simulink model "VIENA_part4"  (R2024b)
settings: Solver=VariableStepAuto  StartTime=0.0  StopTime=t_max  FixedStep=dt  MaxStep=1e-4  RelTol=1e-4
values from neighbouring files (symbols this model uses):
  A = carParameters.frontalArea    [run.m]
  Cd = carParameters.dragCoefficient    [run.m]
  equivalentMass = ((carParameters.Mass) + (totalInertia/(carParameters.wheelRadius^2)))    [run.m]
  fr = carParameters.wheelFriction    [run.m]
  g = 9.81    [run.m]
  lf = 3.23/2    (= 1.615)    [run.m]
  LM = 1.0122e-3    (= 0.0010122)    [run.m]
  LMatrix = [LS 0 LM 0; 0 LS 0 LM; LM 0 LR 0; 0 LM 0 LR]    [run.m]
  lr = 0.06709e-3    (= 6.709e-05)    [run.m]
  LR = lr + LM    (= 0.00107929)    [run.m]
  m = 700 + str2double(mechInput{1})    [run.m]
  maxID = sqrt(2)*Imb    [run.m]
  maxIQ = sqrt(2*Ib^2 - Imb^2)    [run.m]
  maxTorque = 65    [run.m]
  Pp = 2    [run.m]
  psi0 = atan2((x2-x0),(y2-y0))    [run.m]
  rho = carParameters.airDensity    [run.m]
  RLInv = RMatrix/(LMatrix)    [run.m]
  roadAngle = str2double(mechInput{2})*pi/180    [run.m]
  Rr = 2*5.10e-3    (= 0.0102)    [run.m]
  rw = 0.1651    [run.m]
  Steering = FIAT.SteeringController('method','pure pursuit')    [run.m]
  t_sample = 0.1    [run.m]
  x0 = Map.map_points(1,1)    [run.m]
  y0 = Map.map_points(1,2)    [run.m]
libraries: slpidlib x3, simulink_extras x1, spsEdgeDetectorLib x1, simulink x1
settings Model: Creator=João Fernandes  LastModifiedBy=rafae
settings SolverCC: AlgebraicLoopSolver=TrustRegion
settings DataIOCC: ReturnWorkspaceOutputs=off
settings DebuggingCC: UnconnectedInputMsg=warning  UnconnectedOutputMsg=warning  UnconnectedLineMsg=warning  ArithmeticOperatorsInVariantConditions=warning
settings ModelReferenceCC: EnableRefExpFcnMdlSchedulingChecks=on
settings SFSimCC: SimUseLocalCustomCode=off  CustomCodeUndefinedFunction=UseInterfaceOnly
settings RTWCC: RTWUseLocalCustomCode=off  GPUComputeCapability=3.5

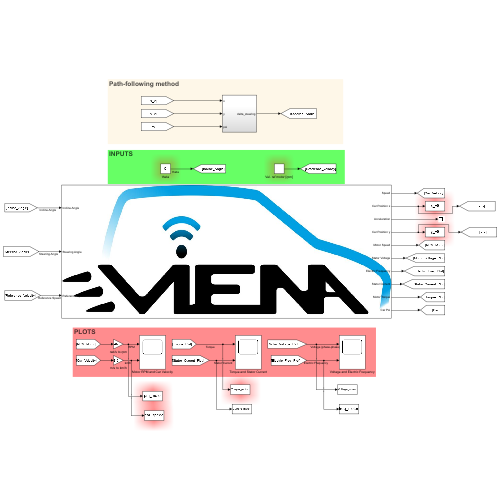
[thumbnail: Simulink's stored preview of the top-level diagram]
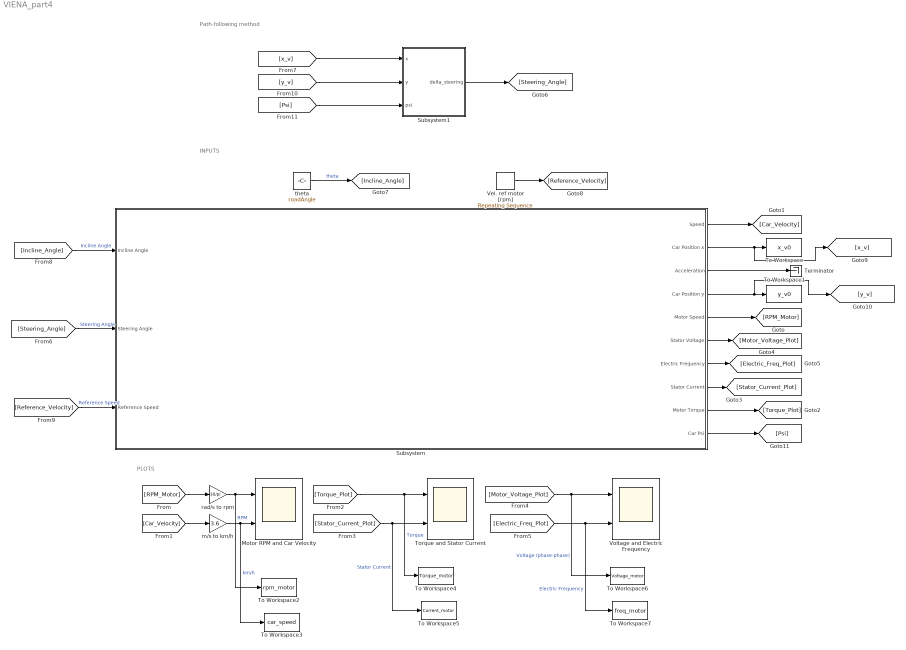
== system VIENA_part4 ==
  note: INPUTS
  note: PLOTS
  note: Path-following method
  Motor RPM and Car Velocity : Scope  NumInputPorts=2
  Subsystem : Subsystem
      mask Display: image('vienalogo.jpg');
  Subsystem1 : Subsystem
  Terminator : Terminator
  To Workspace : ToWorkspace  VariableName=x_v0  SaveFormat=Timeseries  SampleTime=t_sample
  To Workspace1 : ToWorkspace  VariableName=y_v0  SaveFormat=Timeseries  SampleTime=t_sample
  To Workspace2 : ToWorkspace  VariableName=rpm_motor  SaveFormat=Timeseries  SampleTime=t_sample
  To Workspace3 : ToWorkspace  VariableName=car_speed  SaveFormat=Timeseries  SampleTime=t_sample
  To Workspace4 : ToWorkspace  VariableName=Torque_motor  SaveFormat=Timeseries  SampleTime=t_sample
  To Workspace5 : ToWorkspace  VariableName=Current_motor  SaveFormat=Timeseries  SampleTime=-1
  To Workspace6 : ToWorkspace  VariableName=Voltage_motor  SaveFormat=Timeseries  SampleTime=-1
  To Workspace7 : ToWorkspace  VariableName=freq_motor  SaveFormat=Timeseries  SampleTime=-1
  Torque and Stator Current : Scope  NumInputPorts=2
  Vel. ref motor [rpm] : simulink/Sources/Repeating Sequence  rep_seq_t=v_t  rep_seq_y=v_v
  Voltage and Electric Frequency : Scope  NumInputPorts=2
  m/s to km/h : Gain  Gain=3.6
  rad/s to rpm : Gain  Gain=30/pi
  theta : Constant  Value=roadAngle
  wires:
  [RPM_Motor] -> rad/s to rpm/1
  [Car_Velocity] -> m/s to km/h/1
  m/s to km/h/1 -> To Workspace3/1, Motor RPM and Car Velocity/2  "km/h"
  rad/s to rpm/1 -> To Workspace2/1, Motor RPM and Car Velocity/1  "RPM"
  [Torque_Plot] -> To Workspace4/1, Torque and Stator Current/1  "Torque"
  [Stator_Current_Plot] -> To Workspace5/1, Torque and Stator Current/2  "Stator Current"
  [Motor_Voltage_Plot] -> To Workspace6/1, Voltage and Electric Frequency/1  "Voltage (phase-phase)"
  [Electric_Freq_Plot] -> To Workspace7/1, Voltage and Electric Frequency/2  "Electric Frequency"
  theta/1 -> [Incline_Angle]  "theta"
  Vel. ref motor [rpm]/1 -> [Reference_Velocity]
  [Incline_Angle] -> Subsystem/1(Incline Angle)  "Incline Angle"
  [Steering_Angle] -> Subsystem/2(Steering Angle)  "Steering Angle"
  [Reference_Velocity] -> Subsystem/3(Reference Speed)  "Reference Speed"
  Subsystem/1(Speed) -> [Car_Velocity]
  Subsystem/2(Car Position x) -> [x_v], To Workspace/1
  Subsystem/3(Acceleration) -> Terminator/1
  Subsystem/4(Car Position y) -> [y_v], To Workspace1/1
  Subsystem/5(Motor Speed) -> [RPM_Motor]
  Subsystem/6(Stator Voltage) -> [Motor_Voltage_Plot]
  Subsystem/7(Electric Frequency) -> [Electric_Freq_Plot]
  Subsystem/8(Stator Current) -> [Stator_Current_Plot]
  Subsystem/9(Motor Torque) -> [Torque_Plot]
  [x_v] -> Subsystem1/1(x)
  [y_v] -> Subsystem1/2(y)
  Subsystem1/1(delta_steering) -> [Steering_Angle]
  Subsystem/10(Car Psi) -> [Psi]
  [Psi] -> Subsystem1/3(psi)

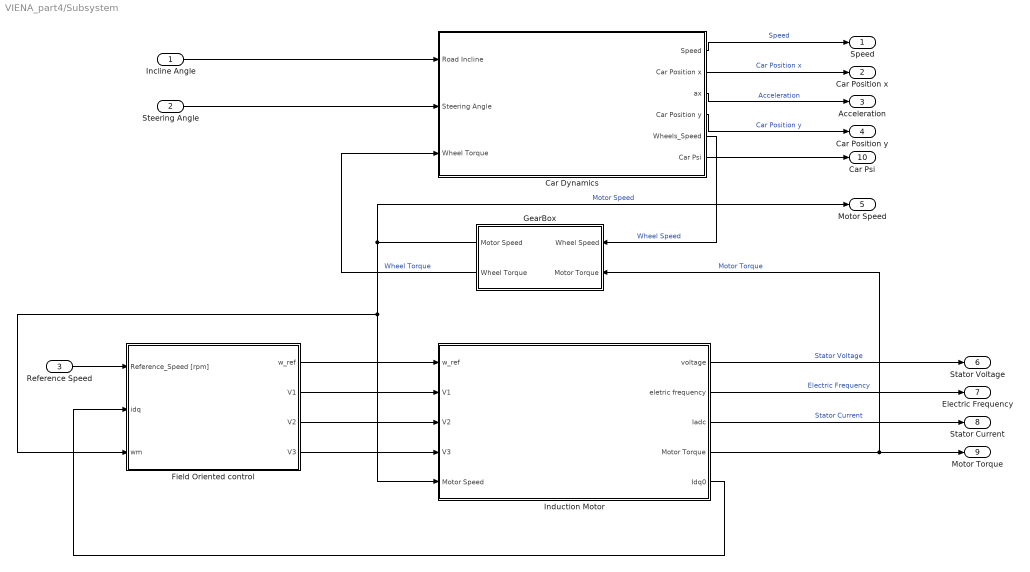
== system VIENA_part4/Subsystem ==
  Incline Angle : Inport
  Steering Angle : Inport  Port=2
  Reference Speed : Inport  Port=3
  Car Dynamics : Subsystem
  "Field Oriented control " : Subsystem
  GearBox : Subsystem
  Induction Motor : Subsystem
  Speed : Outport  VectorParamsAs1DForOutWhenUnconnected=off
  Car Position x : Outport  Port=2  VectorParamsAs1DForOutWhenUnconnected=off
  Acceleration : Outport  Port=3  VectorParamsAs1DForOutWhenUnconnected=off
  Car Position y : Outport  Port=4  VectorParamsAs1DForOutWhenUnconnected=off
  Motor Speed : Outport  Port=5  VectorParamsAs1DForOutWhenUnconnected=off
  Stator Voltage : Outport  Port=6  VectorParamsAs1DForOutWhenUnconnected=off
  Electric Frequency : Outport  Port=7  VectorParamsAs1DForOutWhenUnconnected=off
  Stator Current : Outport  Port=8  VectorParamsAs1DForOutWhenUnconnected=off
  Motor Torque : Outport  Port=9  VectorParamsAs1DForOutWhenUnconnected=off
  Car Psi : Outport  Port=10  VectorParamsAs1DForOutWhenUnconnected=off
  wires:
  GearBox/1("Motor Speed ") -> Induction Motor/5(Motor Speed), "Field Oriented control "/3(wm), Motor Speed/1  "Motor Speed"
  GearBox/2(Wheel Torque) -> Car Dynamics/3(Wheel Torque)  "Wheel Torque"
  Incline Angle/1 -> Car Dynamics/1(Road Incline)
  Induction Motor/1(voltage) -> Stator Voltage/1  "Stator Voltage"
  Car Dynamics/1(Speed) -> Speed/1  "Speed"
  Car Dynamics/5(Wheels_Speed) -> GearBox/1(Wheel Speed)  "Wheel Speed"
  Induction Motor/2(eletric frequency) -> Electric Frequency/1  "Electric Frequency"
  Induction Motor/4(Motor Torque) -> Motor Torque/1, GearBox/2(Motor Torque)  "Motor Torque"
  Car Dynamics/2(Car Position x) -> Car Position x/1  "Car Position x"
  Steering Angle/1 -> Car Dynamics/2(Steering Angle)
  Car Dynamics/4(Car Position y) -> Car Position y/1  "Car Position y"
  Induction Motor/3(Iadc) -> Stator Current/1  "Stator Current"
  Car Dynamics/3(ax) -> Acceleration/1  "Acceleration"
  Car Dynamics/6(Car Psi) -> Car Psi/1
  Reference Speed/1 -> "Field Oriented control "/1(Reference_Speed [rpm])
  "Field Oriented control "/2(V1) -> Induction Motor/2(V1)
  "Field Oriented control "/1(w_ref) -> Induction Motor/1(w_ref)
  "Field Oriented control "/3(V2) -> Induction Motor/3(V2)
  "Field Oriented control "/4(V3) -> Induction Motor/4(V3)
  Induction Motor/5(Idq0) -> "Field Oriented control "/2(idq)

== system VIENA_part4/Subsystem1 ==
  x : Inport
  y : Inport  Port=2
  psi : Inport  Port=3
  Clock : simulink_extras/Flip Flops/Clock  period=dt
  Control steering (with fixed frequency) : Subsystem  TreatAsAtomicUnit=on
  Edge Detector1 : spsEdgeDetectorLib/Edge Detector  model=Rising  ic=0  Ts=0
      settings: LibrarySourceBlock=sps_lib/Control/Edge Detector
  Memory : Memory
  Scope : Scope  NumInputPorts=3
  delta_steering : Outport  VectorParamsAs1DForOutWhenUnconnected=off
  wires:
  Edge Detector1/1 -> Control steering (with fixed frequency)/Enable, Scope/2
  Clock/1 -> Edge Detector1/1
  x/1 -> Control steering (with fixed frequency)/1(x)
  y/1 -> Control steering (with fixed frequency)/2(y)
  psi/1 -> Control steering (with fixed frequency)/3(psi)
  Control steering (with fixed frequency)/1(delta) -> Memory/1, Scope/1
  Memory/1 -> Scope/3, delta_steering/1

== system VIENA_part4/Subsystem/Car Dynamics ==
  Road Incline : Inport
  Steering Angle : Inport  Port=2
  Wheel Torque : Inport  Port=3
  Car Position : Subsystem
  x-simplified model vehicle+wheel : Subsystem
  Speed : Outport  VectorParamsAs1DForOutWhenUnconnected=off
  Car Position x : Outport  Port=2  VectorParamsAs1DForOutWhenUnconnected=off
  ax : Outport  Port=3  VectorParamsAs1DForOutWhenUnconnected=off
  Car Position y : Outport  Port=4  VectorParamsAs1DForOutWhenUnconnected=off
  Wheels_Speed : Outport  Port=5  VectorParamsAs1DForOutWhenUnconnected=off
  Car Psi : Outport  Port=6  VectorParamsAs1DForOutWhenUnconnected=off
  wires:
  Wheel Torque/1 -> x-simplified model vehicle+wheel/1(wheel_Torque)
  x-simplified model vehicle+wheel/1(Speed) -> Speed/1, Car Position/3(Speed)
  x-simplified model vehicle+wheel/2(Acceleration) -> ax/1  "ax"
  Steering Angle/1 -> Car Position/1(Steering Angle)
  Car Position/2(Car Position y) -> Car Position y/1  "Car_Position_y"
  Road Incline/1 -> x-simplified model vehicle+wheel/2(Incline Angle), Car Position/2(Road Incline)
  x-simplified model vehicle+wheel/3(Wheels_Speed) -> Wheels_Speed/1
  Car Position/1(Car Position x) -> Car Position x/1  "Car_Position_x"
  Car Position/3(Car psi) -> Car Psi/1

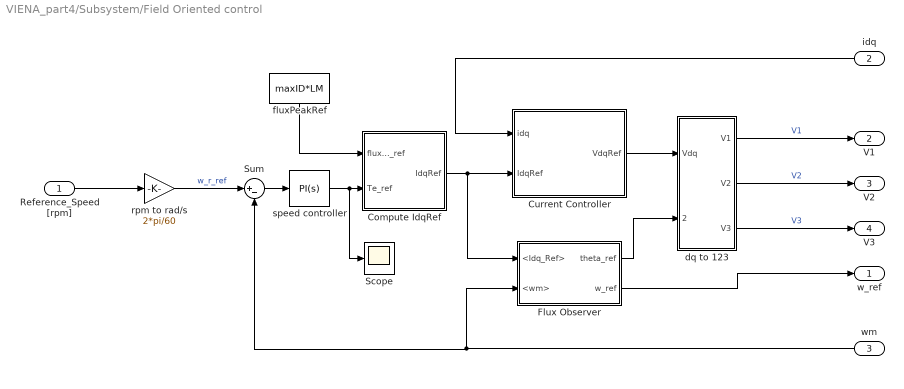
== system VIENA_part4/Subsystem/Field Oriented control  ==
  Reference_Speed [rpm] : Inport
  idq : Inport  Port=2
  wm : Inport  Port=3
  Compute IdqRef : Subsystem
  Current Controller : Subsystem
  Flux Observer : Subsystem
  Scope : Scope
  Sum : Sum  Inputs=|+-
  dq to 123 : Subsystem
  fluxPeakRef : Constant  Value=maxID*LM
  rpm to rad/s : Gain  Gain=2*pi/60
  speed controller : slpidlib/PID Controller  Controller=PI  Form=Parallel  TimeDomain=Continuous-time  UseExternalTs=off  SampleTime=-1  IntegratorMethod=Forward Euler  FilterMethod=Forward Euler  ControllerParametersSource=internal  P=50  I=100  UseKiTs=off  D=0  UseExternalDerivativeSource=off  N=100  UseFilter=on  TunerSelectOption=Transfer Function Based (PID Tuner App)  InitialConditionSource=internal  InitialConditionForIntegrator=0  InitialConditionForFilter=0  DifferentiatorICPrevScaledInput=0  ExternalReset=none  TrackingMode=off  Kt=1  LimitOutput=on  SatLimitsSource=internal  UpperSaturationLimit=maxTorque  LowerSaturationLimit=-maxTorque  LinearizeAsGain=on  AntiWindupMode=back-calculation  Kb=500  LimitIntegrator=off  UpperIntegratorSaturationLimit=inf  LowerIntegratorSaturationLimit=-inf  POutMin=[]  POutMax=[]  IOutMin=[]  IOutMax=[]  DOutMin=[]  DOutMax=[]  NOutMin=[]  NOutMax=[]  SumOutMin=[]  SumOutMax=[]  SaturationOutMin=[]  SaturationOutMax=[]  PParamMin=[]  PParamMax=[]  IParamMin=[]  IParamMax=[]  DParamMin=[]  DParamMax=[]  NParamMin=[]  NParamMax=[]  KbParamMin=[]  KbParamMax=[]  KtParamMin=[]  KtParamMax=[]  KbOutMin=[]  KbOutMax=[]  KtOutMin=[]  KtOutMax=[]  IntegratorOutMin=[]  IntegratorOutMax=[]  FilterOutMin=[]  FilterOutMax=[]  SumI1OutMin=[]  SumI1OutMax=[]  SumI2OutMin=[]  SumI2OutMax=[]  SumI3OutMin=[]  SumI3OutMax=[]  SumI4OutMin=[]  SumI4OutMax=[]  SumDOutMin=[]  SumDOutMax=[]  DifferentiatorOutMin=[]  DifferentiatorOutMax=[]  FilterDiffOutCoefMin=[]  FilterDiffOutCoefMax=[]  ReciprocalOutMin=[]  ReciprocalOutMax=[]  SumDenOutMin=[]  SumDenOutMax=[]  SumNumOutMin=[]  SumNumOutMax=[]  DivideOutMin=[]  DivideOutMax=[]  UdiffTsProdOutMin=[]  UdiffTsProdOutMax=[]  NTsProdOutMin=[]  NTsProdOutMax=[]  UintegralTsProdOutMin=[]  UintegralTsProdOutMax=[]  UngainTsProdOutMin=[]  UngainTsProdOutMax=[]  ClampingZeroOutDataTypeStr=Inherit: Inherit via back propagation  ClampingZeroOutMin=[]  ClampingZeroOutMax=[]  FilterDenConstantOutDataTypeStr=Inherit: Inherit via back propagation  FilterDenConstantOutMin=[]  FilterDenConstantOutMax=[]  PCopyOutDataTypeStr=Inherit: Inherit via back propagation  PCopyOutMin=[]  PCopyOutMax=[]  NCopyOutDataTypeStr=Inherit: Inherit via back propagation  NCopyOutMin=[]  NCopyOutMax=[]  IntegratorContinuousStateAttributes=''  IntegratorStateMustResolveToSignalObject=off  IntegratorRTWStateStorageClass=Auto  FilterContinuousStateAttributes=''  FilterStateMustResolveToSignalObject=off  FilterRTWStateStorageClass=Auto  ParallelPVariant=InternalParameters  IdealPVariant=Disabled  IVariant=InternalParameters  DVariant=Disabled  IntegratorVariant=Continuous  SatVariant=Enabled  AWVariant=BackCalculation  PCopyVariant=Disabled  TRVariant=Disabled  FdbkBlocksVariant=Forward  IdealPFdbkVariant=Disabled  SatFdbkVariant=Disabled  DerivativeFilterVariant=Disabled  NVariant=Disabled  NCopyVariant=Disabled_SignalSpec  FilterICVariant=Disabled  IntegratorICVariant=InternalICs  ExternalResetVariant=Disabled  TRSumVariant=Passthrough  SumFdbkVariant=Disabled  SumVariant=Sum_PI  TsampFilterVariant=InternalTs  TsampNgainVariant=Passthrough  TsampIntegralVariant=Disabled_SignalSpec  ExternalSaturationOutDataTypeStr=Inherit: Same as second input  DerivativeSourceVariant=Disabled  PreIntVariant=InternalPreInt
  w_ref : Outport  VectorParamsAs1DForOutWhenUnconnected=off
  V1 : Outport  Port=2  VectorParamsAs1DForOutWhenUnconnected=off
  V2 : Outport  Port=3  VectorParamsAs1DForOutWhenUnconnected=off
  V3 : Outport  Port=4  VectorParamsAs1DForOutWhenUnconnected=off
  wires:
  wm/1 -> Sum/2, Flux Observer/2(<wm>)
  Current Controller/1(VdqRef) -> dq to 123/1(Vdq)
  idq/1 -> Current Controller/1(idq)
  Flux Observer/2(w_ref) -> w_ref/1
  Compute IdqRef/1(IdqRef) -> Flux Observer/1(<Idq_Ref>), Current Controller/2(IdqRef)
  Sum/1 -> speed controller/1
  fluxPeakRef/1 -> Compute IdqRef/1(fluxdR_ref)
  Flux Observer/1(theta_ref) -> dq to 123/2(theta_ref)
  dq to 123/3(V3) -> V3/1  "V3"
  dq to 123/1(V1) -> V1/1  "V1"
  speed controller/1 -> Scope/1, Compute IdqRef/2(Te_ref)
  dq to 123/2(V2) -> V2/1  "V2"
  Reference_Speed [rpm]/1 -> rpm to rad/s/1
  rpm to rad/s/1 -> Sum/1  "w_r_ref"

== system VIENA_part4/Subsystem/GearBox ==
  Wheel Speed : Inport
  Motor Torque : Inport  Port=2
  Gain : Gain  Gain=8
  Gain1 : Gain  Gain=8
  "Motor Speed " : Outport  VectorParamsAs1DForOutWhenUnconnected=off
  Wheel Torque : Outport  Port=2  VectorParamsAs1DForOutWhenUnconnected=off
  wires:
  Wheel Speed/1 -> Gain/1
  Gain/1 -> "Motor Speed "/1
  Motor Torque/1 -> Gain1/1
  Gain1/1 -> Wheel Torque/1

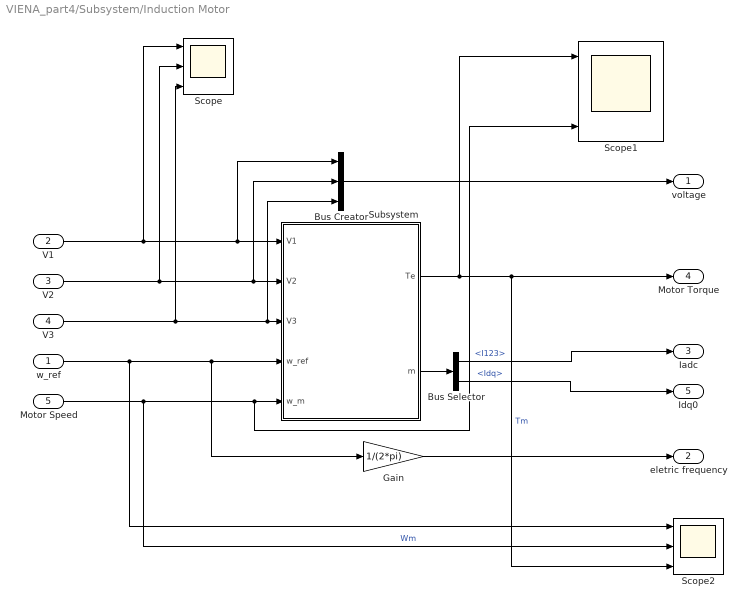
== system VIENA_part4/Subsystem/Induction Motor ==
  w_ref : Inport
  V1 : Inport  Port=2
  V2 : Inport  Port=3
  V3 : Inport  Port=4
  Motor Speed : Inport  Port=5
  Bus Creator : BusCreator  Inputs=3
  Bus Selector : BusSelector  OutputSignals=I123,Idq
  Gain : Gain  Gain=1/(2*pi)
  Scope : Scope  NumInputPorts=3
  Scope1 : Scope  NumInputPorts=3
  Scope2 : Scope  NumInputPorts=3
  Subsystem : Subsystem
  voltage : Outport  VectorParamsAs1DForOutWhenUnconnected=off
  eletric frequency : Outport  Port=2  VectorParamsAs1DForOutWhenUnconnected=off
  Iadc : Outport  Port=3  VectorParamsAs1DForOutWhenUnconnected=off
  Motor Torque : Outport  Port=4  VectorParamsAs1DForOutWhenUnconnected=off
  Idq0 : Outport  Port=5  VectorParamsAs1DForOutWhenUnconnected=off
  wires:
  Subsystem/1(Te) -> Scope1/1, Scope2/3, Motor Torque/1  "Tm"
  Motor Speed/1 -> Scope2/2, Scope1/3, Subsystem/5(w_m)  "Wm"
  Subsystem/2(m) -> Bus Selector/1
  Bus Selector/1 -> Iadc/1  "<I123>"
  V3/1 -> Scope/3, Bus Creator/3, Subsystem/3(V3)
  V2/1 -> Bus Creator/2, Subsystem/2(V2), Scope/2
  V1/1 -> Bus Creator/1, Subsystem/1(V1), Scope/1
  w_ref/1 -> Scope2/1, Gain/1, Subsystem/4(w_ref)
  Gain/1 -> eletric frequency/1
  Bus Creator/1 -> voltage/1
  Bus Selector/2 -> Idq0/1  "<Idq>"

== system VIENA_part4/Subsystem1/Control steering (with fixed frequency) ==
  x : Inport
  y : Inport  Port=2
  psi : Inport  Port=3
  Enable : EnablePort
  Constant1 : Constant  Value=Steering.map_points  VectorParams1D=off
  Saturation : Saturate  UpperLimit=28*pi/180  LowerLimit=-28*pi/180
  Stop Simulation : Stop
  compute diff angle : MATLAB Function  TreatAsAtomicUnit=on
  cria look_ahead : MATLAB Function  TreatAsAtomicUnit=on
  find index : MATLAB Function  TreatAsAtomicUnit=on
  delta : Outport  VectorParamsAs1DForOutWhenUnconnected=off
  wires:
  x/1 -> compute diff angle/2(x), find index/2(x)
  y/1 -> compute diff angle/3("y "), find index/3("y ")
  Constant1/1 -> cria look_ahead/1(map), find index/1(u)
  find index/1(y) -> cria look_ahead/2(path_index)
  cria look_ahead/2(y2) -> Stop Simulation/1
  compute diff angle/1(y) -> Saturation/1
  cria look_ahead/1(y1) -> compute diff angle/1(zone)
  psi/1 -> compute diff angle/4(psi)
  Saturation/1 -> delta/1

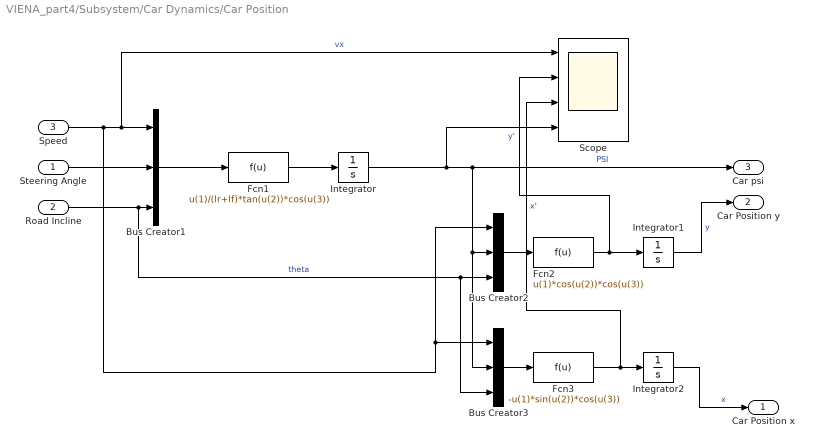
== system VIENA_part4/Subsystem/Car Dynamics/Car Position ==
  Steering Angle : Inport
  Road Incline : Inport  Port=2
  Speed : Inport  Port=3
  Bus Creator1 : BusCreator  Inputs=3
  Bus Creator2 : BusCreator  Inputs=3
  Bus Creator3 : BusCreator  Inputs=3
  Fcn1 : Fcn  Expr=u(1)/(lr+lf)*tan(u(2))*cos(u(3))
  Fcn2 : Fcn  Expr=u(1)*cos(u(2))*cos(u(3))
  Fcn3 : Fcn  Expr=-u(1)*sin(u(2))*cos(u(3))
  Integrator : Integrator  InitialCondition=psi0
  Integrator1 : Integrator  InitialCondition=y0
  Integrator2 : Integrator  InitialCondition=x0
  Scope : Scope  NumInputPorts=4
  Car Position x : Outport  VectorParamsAs1DForOutWhenUnconnected=off
  Car Position y : Outport  Port=2  VectorParamsAs1DForOutWhenUnconnected=off
  Car psi : Outport  Port=3  VectorParamsAs1DForOutWhenUnconnected=off
  wires:
  Integrator1/1 -> Car Position y/1  "y"
  Integrator2/1 -> Car Position x/1  "x"
  Road Incline/1 -> Bus Creator3/3, Bus Creator2/3, Bus Creator1/3  "theta"
  Bus Creator1/1 -> Fcn1/1
  Fcn1/1 -> Integrator/1
  Bus Creator2/1 -> Fcn2/1
  Speed/1 -> Bus Creator2/1, Bus Creator3/1, Scope/1, Bus Creator1/1  "vx"
  Fcn2/1 -> Scope/2, Integrator1/1  "y'"
  Fcn3/1 -> Scope/3, Integrator2/1  "x'"
  Integrator/1 -> Car psi/1, Bus Creator3/2, Bus Creator2/2, Scope/4  "PSI"
  Bus Creator3/1 -> Fcn3/1
  Steering Angle/1 -> Bus Creator1/2

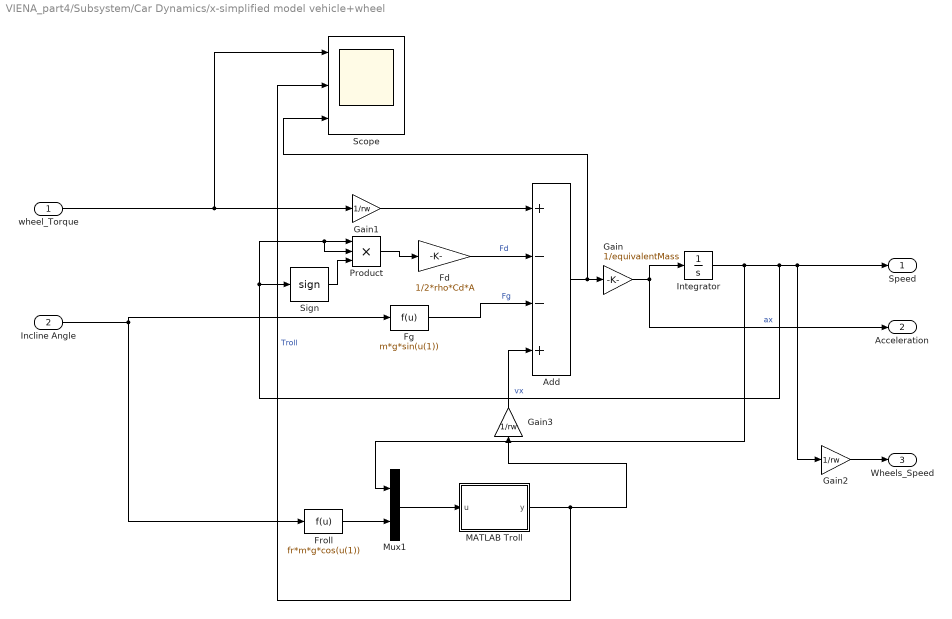
== system VIENA_part4/Subsystem/Car Dynamics/x-simplified model vehicle+wheel ==
  wheel_Torque : Inport
  Incline Angle : Inport  Port=2
  Add : Sum  Inputs=+--+
  Fd : Gain  Gain=1/2*rho*Cd*A
  Fg : Fcn  Expr=m*g*sin(u(1))
  Froll : Fcn  Expr=fr*m*g*cos(u(1))
  Gain : Gain  Gain=1/equivalentMass
  Gain1 : Gain  Gain=1/rw
  Gain2 : Gain  Gain=1/rw
  Gain3 : Gain  Gain=1/rw
  Integrator : Integrator
  MATLAB Troll : MATLAB Function  TreatAsAtomicUnit=on
  Mux1 : Mux  Inputs=2
  Product : Product  Inputs=3
  Scope : Scope  NumInputPorts=3
  Sign : Signum
  Speed : Outport  VectorParamsAs1DForOutWhenUnconnected=off
  Acceleration : Outport  Port=2  VectorParamsAs1DForOutWhenUnconnected=off
  Wheels_Speed : Outport  Port=3  VectorParamsAs1DForOutWhenUnconnected=off
  wires:
  Product/1 -> Fd/1
  Incline Angle/1 -> Froll/1, Fg/1
  Fg/1 -> Add/3  "Fg"
  Add/1 -> Scope/3, Gain/1
  Gain/1 -> Integrator/1, Acceleration/1  "ax"
  Fd/1 -> Add/2  "Fd"
  Integrator/1 -> Mux1/1, Gain2/1, Speed/1, Sign/1, Product/2, Product/1  "vx"
  Sign/1 -> Product/3
  Gain1/1 -> Add/1
  Gain2/1 -> Wheels_Speed/1
  wheel_Torque/1 -> Scope/1, Gain1/1
  Froll/1 -> Mux1/2
  Mux1/1 -> MATLAB Troll/1(u)
  MATLAB Troll/1(y) -> Scope/2, Gain3/1  "Troll"
  Gain3/1 -> Add/4

== system VIENA_part4/Subsystem/Field Oriented control /Compute IdqRef ==
  fluxdR_ref : Inport
  Te_ref : Inport  Port=2
  Fcn : Fcn  Expr=u(2)/(3/2*Pp*(LM/LR)*u(1))
  Gain : Gain  Gain=1/LM
  Mux : Mux  Inputs=2
  Mux1 : Mux  Inputs=2
  Saturation : Saturate  UpperLimit=maxID  LowerLimit=-maxID
  Saturation1 : Saturate  UpperLimit=maxIQ  LowerLimit=-maxIQ
  IdqRef : Outport  VectorParamsAs1DForOutWhenUnconnected=off
  wires:
  fluxdR_ref/1 -> Mux/1, Gain/1
  Mux/1 -> Fcn/1
  Fcn/1 -> Saturation1/1
  Gain/1 -> Saturation/1
  Mux1/1 -> IdqRef/1
  Te_ref/1 -> Mux/2
  Saturation/1 -> Mux1/1  "id"
  Saturation1/1 -> Mux1/2  "iq"

== system VIENA_part4/Subsystem/Field Oriented control /Current Controller ==
  idq : Inport
  IdqRef : Inport  Port=2
  Demux : Demux  Outputs=2
  Mux : Mux  Inputs=2
  PID Controller : slpidlib/PID Controller  Controller=PI  Form=Parallel  TimeDomain=Continuous-time  UseExternalTs=off  SampleTime=-1  IntegratorMethod=Forward Euler  FilterMethod=Forward Euler  ControllerParametersSource=internal  P=5  I=100  UseKiTs=off  D=0  UseExternalDerivativeSource=off  N=100  UseFilter=on  TunerSelectOption=Transfer Function Based (PID Tuner App)  InitialConditionSource=internal  InitialConditionForIntegrator=0  InitialConditionForFilter=0  DifferentiatorICPrevScaledInput=0  ExternalReset=none  TrackingMode=off  Kt=1  LimitOutput=on  SatLimitsSource=internal  UpperSaturationLimit=600  LowerSaturationLimit=-600  LinearizeAsGain=on  AntiWindupMode=back-calculation  Kb=1  LimitIntegrator=off  UpperIntegratorSaturationLimit=inf  LowerIntegratorSaturationLimit=-inf  POutMin=[]  POutMax=[]  IOutMin=[]  IOutMax=[]  DOutMin=[]  DOutMax=[]  NOutMin=[]  NOutMax=[]  SumOutMin=[]  SumOutMax=[]  SaturationOutMin=[]  SaturationOutMax=[]  PParamMin=[]  PParamMax=[]  IParamMin=[]  IParamMax=[]  DParamMin=[]  DParamMax=[]  NParamMin=[]  NParamMax=[]  KbParamMin=[]  KbParamMax=[]  KtParamMin=[]  KtParamMax=[]  KbOutMin=[]  KbOutMax=[]  KtOutMin=[]  KtOutMax=[]  IntegratorOutMin=[]  IntegratorOutMax=[]  FilterOutMin=[]  FilterOutMax=[]  SumI1OutMin=[]  SumI1OutMax=[]  SumI2OutMin=[]  SumI2OutMax=[]  SumI3OutMin=[]  SumI3OutMax=[]  SumI4OutMin=[]  SumI4OutMax=[]  SumDOutMin=[]  SumDOutMax=[]  DifferentiatorOutMin=[]  DifferentiatorOutMax=[]  FilterDiffOutCoefMin=[]  FilterDiffOutCoefMax=[]  ReciprocalOutMin=[]  ReciprocalOutMax=[]  SumDenOutMin=[]  SumDenOutMax=[]  SumNumOutMin=[]  SumNumOutMax=[]  DivideOutMin=[]  DivideOutMax=[]  UdiffTsProdOutMin=[]  UdiffTsProdOutMax=[]  NTsProdOutMin=[]  NTsProdOutMax=[]  UintegralTsProdOutMin=[]  UintegralTsProdOutMax=[]  UngainTsProdOutMin=[]  UngainTsProdOutMax=[]  ClampingZeroOutDataTypeStr=Inherit: Inherit via back propagation  ClampingZeroOutMin=[]  ClampingZeroOutMax=[]  FilterDenConstantOutDataTypeStr=Inherit: Inherit via back propagation  FilterDenConstantOutMin=[]  FilterDenConstantOutMax=[]  PCopyOutDataTypeStr=Inherit: Inherit via back propagation  PCopyOutMin=[]  PCopyOutMax=[]  NCopyOutDataTypeStr=Inherit: Inherit via back propagation  NCopyOutMin=[]  NCopyOutMax=[]  IntegratorContinuousStateAttributes=''  IntegratorStateMustResolveToSignalObject=off  IntegratorRTWStateStorageClass=Auto  FilterContinuousStateAttributes=''  FilterStateMustResolveToSignalObject=off  FilterRTWStateStorageClass=Auto  ParallelPVariant=InternalParameters  IdealPVariant=Disabled  IVariant=InternalParameters  DVariant=Disabled  IntegratorVariant=Continuous  SatVariant=Enabled  AWVariant=BackCalculation  PCopyVariant=Disabled  TRVariant=Disabled  FdbkBlocksVariant=Forward  IdealPFdbkVariant=Disabled  SatFdbkVariant=Disabled  DerivativeFilterVariant=Disabled  NVariant=Disabled  NCopyVariant=Disabled_SignalSpec  FilterICVariant=Disabled  IntegratorICVariant=InternalICs  ExternalResetVariant=Disabled  TRSumVariant=Passthrough  SumFdbkVariant=Disabled  SumVariant=Sum_PI  TsampFilterVariant=InternalTs  TsampNgainVariant=Passthrough  TsampIntegralVariant=Disabled_SignalSpec  ExternalSaturationOutDataTypeStr=Inherit: Same as second input  DerivativeSourceVariant=Disabled  PreIntVariant=InternalPreInt
  PID Controller1 : slpidlib/PID Controller  Controller=PI  Form=Parallel  TimeDomain=Continuous-time  UseExternalTs=off  SampleTime=-1  IntegratorMethod=Forward Euler  FilterMethod=Forward Euler  ControllerParametersSource=internal  P=5  I=100  UseKiTs=off  D=0  UseExternalDerivativeSource=off  N=100  UseFilter=on  TunerSelectOption=Transfer Function Based (PID Tuner App)  InitialConditionSource=internal  InitialConditionForIntegrator=0  InitialConditionForFilter=0  DifferentiatorICPrevScaledInput=0  ExternalReset=none  TrackingMode=off  Kt=1  LimitOutput=on  SatLimitsSource=internal  UpperSaturationLimit=600  LowerSaturationLimit=-600  LinearizeAsGain=on  AntiWindupMode=back-calculation  Kb=1  LimitIntegrator=off  UpperIntegratorSaturationLimit=inf  LowerIntegratorSaturationLimit=-inf  POutMin=[]  POutMax=[]  IOutMin=[]  IOutMax=[]  DOutMin=[]  DOutMax=[]  NOutMin=[]  NOutMax=[]  SumOutMin=[]  SumOutMax=[]  SaturationOutMin=[]  SaturationOutMax=[]  PParamMin=[]  PParamMax=[]  IParamMin=[]  IParamMax=[]  DParamMin=[]  DParamMax=[]  NParamMin=[]  NParamMax=[]  KbParamMin=[]  KbParamMax=[]  KtParamMin=[]  KtParamMax=[]  KbOutMin=[]  KbOutMax=[]  KtOutMin=[]  KtOutMax=[]  IntegratorOutMin=[]  IntegratorOutMax=[]  FilterOutMin=[]  FilterOutMax=[]  SumI1OutMin=[]  SumI1OutMax=[]  SumI2OutMin=[]  SumI2OutMax=[]  SumI3OutMin=[]  SumI3OutMax=[]  SumI4OutMin=[]  SumI4OutMax=[]  SumDOutMin=[]  SumDOutMax=[]  DifferentiatorOutMin=[]  DifferentiatorOutMax=[]  FilterDiffOutCoefMin=[]  FilterDiffOutCoefMax=[]  ReciprocalOutMin=[]  ReciprocalOutMax=[]  SumDenOutMin=[]  SumDenOutMax=[]  SumNumOutMin=[]  SumNumOutMax=[]  DivideOutMin=[]  DivideOutMax=[]  UdiffTsProdOutMin=[]  UdiffTsProdOutMax=[]  NTsProdOutMin=[]  NTsProdOutMax=[]  UintegralTsProdOutMin=[]  UintegralTsProdOutMax=[]  UngainTsProdOutMin=[]  UngainTsProdOutMax=[]  ClampingZeroOutDataTypeStr=Inherit: Inherit via back propagation  ClampingZeroOutMin=[]  ClampingZeroOutMax=[]  FilterDenConstantOutDataTypeStr=Inherit: Inherit via back propagation  FilterDenConstantOutMin=[]  FilterDenConstantOutMax=[]  PCopyOutDataTypeStr=Inherit: Inherit via back propagation  PCopyOutMin=[]  PCopyOutMax=[]  NCopyOutDataTypeStr=Inherit: Inherit via back propagation  NCopyOutMin=[]  NCopyOutMax=[]  IntegratorContinuousStateAttributes=''  IntegratorStateMustResolveToSignalObject=off  IntegratorRTWStateStorageClass=Auto  FilterContinuousStateAttributes=''  FilterStateMustResolveToSignalObject=off  FilterRTWStateStorageClass=Auto  ParallelPVariant=InternalParameters  IdealPVariant=Disabled  IVariant=InternalParameters  DVariant=Disabled  IntegratorVariant=Continuous  SatVariant=Enabled  AWVariant=BackCalculation  PCopyVariant=Disabled  TRVariant=Disabled  FdbkBlocksVariant=Forward  IdealPFdbkVariant=Disabled  SatFdbkVariant=Disabled  DerivativeFilterVariant=Disabled  NVariant=Disabled  NCopyVariant=Disabled_SignalSpec  FilterICVariant=Disabled  IntegratorICVariant=InternalICs  ExternalResetVariant=Disabled  TRSumVariant=Passthrough  SumFdbkVariant=Disabled  SumVariant=Sum_PI  TsampFilterVariant=InternalTs  TsampNgainVariant=Passthrough  TsampIntegralVariant=Disabled_SignalSpec  ExternalSaturationOutDataTypeStr=Inherit: Same as second input  DerivativeSourceVariant=Disabled  PreIntVariant=InternalPreInt
  Scope2 : Scope  NumInputPorts=2
  Sum1 : Sum  Inputs=+-
  VdqRef : Outport  VectorParamsAs1DForOutWhenUnconnected=off
  wires:
  IdqRef/1 -> Scope2/1, Sum1/1
  idq/1 -> Sum1/2
  PID Controller/1 -> Mux/1  "PI"
  Sum1/1 -> Scope2/2, Demux/1  "error"
  Demux/1 -> PID Controller/1
  Demux/2 -> PID Controller1/1
  PID Controller1/1 -> Mux/2
  Mux/1 -> VdqRef/1

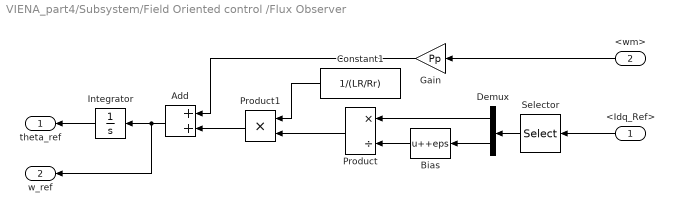
== system VIENA_part4/Subsystem/Field Oriented control /Flux Observer ==
  <Idq_Ref> : Inport
  <wm> : Inport  Port=2
  Add : Sum  Inputs=2
  Bias : Bias  Bias=+eps  SaturateOnIntegerOverflow=off
  Constant1 : Constant  Value=1/(LR/Rr)
  Demux : Demux  Outputs=2
  Gain : Gain  Gain=Pp
  Integrator : Integrator
  Product : Product  Inputs=*/
  Product1 : Product
  Selector : Selector  InputPortWidth=2  IndexOptions=Index vector (dialog)  Indices=[2 1]  OutputSizes=1
  theta_ref : Outport  VectorParamsAs1DForOutWhenUnconnected=off
  w_ref : Outport  Port=2  VectorParamsAs1DForOutWhenUnconnected=off
  wires:
  Demux/1 -> Product/1
  <wm>/1 -> Gain/1
  Constant1/1 -> Product1/1
  Selector/1 -> Demux/1
  Product1/1 -> Add/2
  Product/1 -> Product1/2
  <Idq_Ref>/1 -> Selector/1
  Add/1 -> w_ref/1, Integrator/1
  Bias/1 -> Product/2
  Demux/2 -> Bias/1
  Integrator/1 -> theta_ref/1
  Gain/1 -> Add/1

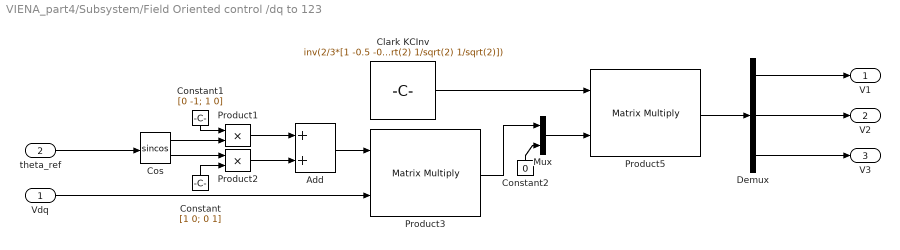
== system VIENA_part4/Subsystem/Field Oriented control /dq to 123 ==
  Vdq : Inport
  theta_ref : Inport  Port=2
  Add : Sum
  Clark KCInv : Constant  Value=inv(2/3*[1 -0.5 -0.5; 0 sqrt(3)/2 -sqrt(3)/2; 1/sqrt(2) 1/sqrt(2) 1/sqrt(2)])
  Constant : Constant  Value=[1 0; 0 1]
  Constant1 : Constant  Value=[0 -1; 1 0]
  Constant2 : Constant  Value=0
  Cos : Trigonometry  Operator=sincos
  Demux : Demux  Outputs=3
  Mux : Mux  Inputs=2
  Product1 : Product
  Product2 : Product
  Product3 : Product  Multiplication=Matrix(*)
  Product5 : Product  Multiplication=Matrix(*)
  V1 : Outport  VectorParamsAs1DForOutWhenUnconnected=off
  V2 : Outport  Port=2  VectorParamsAs1DForOutWhenUnconnected=off
  V3 : Outport  Port=3  VectorParamsAs1DForOutWhenUnconnected=off
  wires:
  Cos/1 -> Product1/2
  Constant1/1 -> Product1/1
  Product2/1 -> Add/2
  Cos/2 -> Product2/1
  Product1/1 -> Add/1
  Constant/1 -> Product2/2
  Add/1 -> Product3/1
  Product3/1 -> Mux/1
  Clark KCInv/1 -> Product5/1
  Mux/1 -> Product5/2
  Constant2/1 -> Mux/2
  Vdq/1 -> Product3/2
  Demux/1 -> V1/1
  Demux/2 -> V2/1
  Demux/3 -> V3/1
  Product5/1 -> Demux/1
  theta_ref/1 -> Cos/1

== system VIENA_part4/Subsystem/Induction Motor/Subsystem ==
  note: V1 - phase-to-neutral voltage of phase 1 [V]
      | V2 - phase-to-neutral voltage of phase 2 [V]
      | V3 - phase-to-neutral voltage of phase 3 [V]
      | w_ref - reference of dq transformation (synchornous electric speed in this case = 2*pi*f) [rad/s]
      | w_m - motor angular speed [rad/s]
  V1 : Inport
  V2 : Inport  Port=2
  V3 : Inport  Port=3
  w_ref : Inport  Port=4
  w_m : Inport  Port=5
  Induction Machine Model : Subsystem
  Te : Outport  VectorParamsAs1DForOutWhenUnconnected=off
  m : Outport  Port=2  VectorParamsAs1DForOutWhenUnconnected=off
  wires:
  Induction Machine Model/1(m) -> m/1
  w_ref/1 -> Induction Machine Model/5(w_ref)
  V1/1 -> Induction Machine Model/2(V1)
  Induction Machine Model/2(Te) -> Te/1
  V2/1 -> Induction Machine Model/3(V2)
  V3/1 -> Induction Machine Model/4(V3)
  w_m/1 -> Induction Machine Model/1(wm)

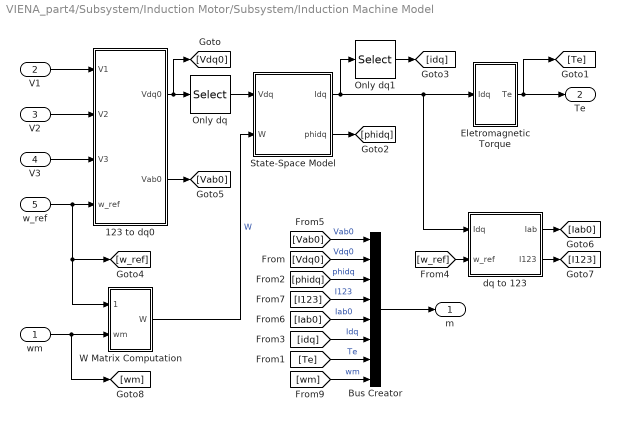
== system VIENA_part4/Subsystem/Induction Motor/Subsystem/Induction Machine Model ==
  wm : Inport
  V1 : Inport  Port=2
  V2 : Inport  Port=3
  V3 : Inport  Port=4
  w_ref : Inport  Port=5
  123 to dq0 : Subsystem
  Bus Creator : BusCreator  Inputs=8
  Eletromagnetic Torque : Subsystem
  Only dq : Selector  InputPortWidth=3  IndexOptions=Index vector (dialog)  Indices=[1 2]  OutputSizes=1
  Only dq1 : Selector  InputPortWidth=4  IndexOptions=Index vector (dialog)  Indices=[1 2]  OutputSizes=1
  State-Space Model : Subsystem
  W Matrix Computation : Subsystem
  dq to 123 : Subsystem
  m : Outport  VectorParamsAs1DForOutWhenUnconnected=off
  Te : Outport  Port=2  VectorParamsAs1DForOutWhenUnconnected=off
  wires:
  123 to dq0/1(Vdq0) -> Only dq/1, [Vdq0]
  V3/1 -> 123 to dq0/3(V3)
  V2/1 -> 123 to dq0/2(V2)
  wm/1 -> [wm], W Matrix Computation/2(wm)
  123 to dq0/2(Vab0) -> [Vab0]
  W Matrix Computation/1(W) -> State-Space Model/2(W)  "W"
  Only dq/1 -> State-Space Model/1(Vdq)
  Eletromagnetic Torque/1(Te) -> Te/1, [Te]
  V1/1 -> 123 to dq0/1(V1)
  State-Space Model/1(Idq) -> dq to 123/1(Idq), Eletromagnetic Torque/1(Idq), Only dq1/1
  [w_ref] -> dq to 123/2(w_ref)
  State-Space Model/2(phidq) -> [phidq]
  dq to 123/1(Iab) -> [Iab0]
  dq to 123/2(I123) -> [I123]
  [Vab0] -> Bus Creator/1  "Vab0"
  [Vdq0] -> Bus Creator/2  "Vdq0"
  [phidq] -> Bus Creator/3  "phidq"
  [I123] -> Bus Creator/4  "I123"
  [Iab0] -> Bus Creator/5  "Iab0"
  [idq] -> Bus Creator/6  "Idq"
  [Te] -> Bus Creator/7  "Te"
  Bus Creator/1 -> m/1
  Only dq1/1 -> [idq]
  w_ref/1 -> 123 to dq0/4(w_ref), W Matrix Computation/1(w_ref), [w_ref]
  [wm] -> Bus Creator/8  "wm"

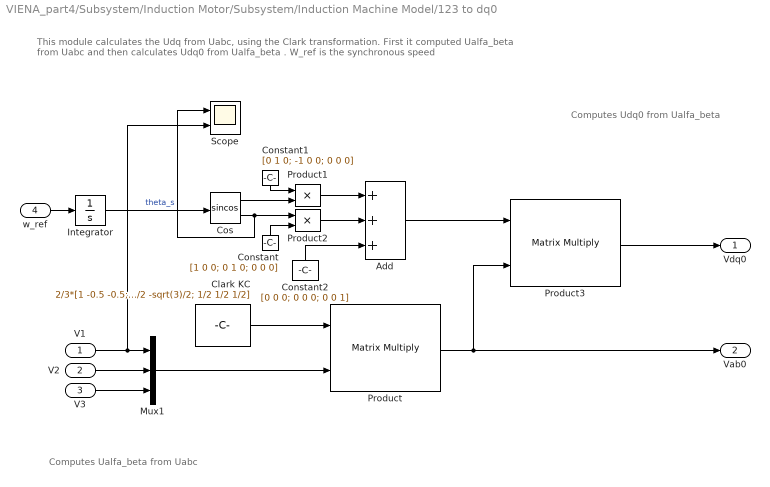
== system VIENA_part4/Subsystem/Induction Motor/Subsystem/Induction Machine Model/123 to dq0 ==
  note: Computes Ualfa_beta from Uabc
  note: This module calculates the Udq from Uabc, using the Clark transformation.
      | First it computed Ualfa_beta from Uabc and then calculates Udq0 from Ualfa_beta .
      | W_ref is the synchronous speed
  note: Computes Udq0 from Ualfa_beta
  V1 : Inport
  V2 : Inport  Port=2
  V3 : Inport  Port=3
  w_ref : Inport  Port=4
  Add : Sum  Inputs=+++
  Clark KC : Constant  Value=2/3*[1 -0.5 -0.5; 0 sqrt(3)/2 -sqrt(3)/2; 1/2 1/2 1/2]
  Constant : Constant  Value=[1 0 0; 0 1 0; 0 0 0]
  Constant1 : Constant  Value=[0 1 0; -1 0 0; 0 0 0]
  Constant2 : Constant  Value=[0 0 0; 0 0 0; 0 0 1]
  Cos : Trigonometry  Operator=sincos
  Integrator : Integrator
  Mux1 : Mux  Inputs=3
  Product : Product  Multiplication=Matrix(*)
  Product1 : Product
  Product2 : Product
  Product3 : Product  Multiplication=Matrix(*)
  Scope : Scope  NumInputPorts=2
  Vdq0 : Outport  VectorParamsAs1DForOutWhenUnconnected=off
  Vab0 : Outport  Port=2  VectorParamsAs1DForOutWhenUnconnected=off
  wires:
  Clark KC/1 -> Product/1
  Mux1/1 -> Product/2
  Product/1 -> Product3/2, Vab0/1
  Integrator/1 -> Cos/1  "theta_s"
  Cos/1 -> Product1/2
  Constant1/1 -> Product1/1
  Cos/2 -> Scope/1, Product2/1
  Constant/1 -> Product2/2
  Product1/1 -> Add/1
  Product2/1 -> Add/2
  Add/1 -> Product3/1
  Product3/1 -> Vdq0/1
  w_ref/1 -> Integrator/1
  Constant2/1 -> Add/3
  V2/1 -> Mux1/2
  V3/1 -> Mux1/3
  V1/1 -> Mux1/1, Scope/2

== system VIENA_part4/Subsystem/Induction Motor/Subsystem/Induction Machine Model/Eletromagnetic Torque ==
  Idq : Inport
  Constant : Constant  Value=3/2*LM*Pp
  Demux1 : Demux  Outputs=2
  Product : Product
  Product1 : Product  Inputs=1
  Product2 : Product  Inputs=1
  Selector : Selector  InputPortWidth=4  IndexOptions=Index vector (dialog)  Indices=[2 3 1 4]  OutputSizes=1
  Sum : Sum  Inputs=+-
  Te : Outport  VectorParamsAs1DForOutWhenUnconnected=off
  wires:
  Sum/1 -> Product/1
  Product1/1 -> Sum/1
  Demux1/1 -> Product1/1
  Product2/1 -> Sum/2
  Constant/1 -> Product/2
  Demux1/2 -> Product2/1
  Product/1 -> Te/1
  Idq/1 -> Selector/1
  Selector/1 -> Demux1/1

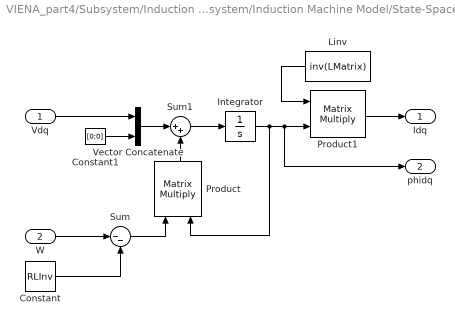
== system VIENA_part4/Subsystem/Induction Motor/Subsystem/Induction Machine Model/State-Space Model ==
  Vdq : Inport
  W : Inport  Port=2
  Constant : Constant  Value=RLInv  VectorParams1D=off
  Constant1 : Constant  Value=[0;0]
  Integrator : Integrator
  Linv : Constant  Value=inv(LMatrix)  VectorParams1D=off
  Product : Product  Multiplication=Matrix(*)
  Product1 : Product  Multiplication=Matrix(*)
  Sum : Sum  Inputs=|--
  Sum1 : Sum  Inputs=|++
  Vector Concatenate : Concatenate
  Idq : Outport  VectorParamsAs1DForOutWhenUnconnected=off
  phidq : Outport  Port=2  VectorParamsAs1DForOutWhenUnconnected=off
  wires:
  W/1 -> Sum/1
  Product/1 -> Sum1/2
  Constant/1 -> Sum/2
  Integrator/1 -> phidq/1, Product1/2, Product/2
  Product1/1 -> Idq/1
  Sum1/1 -> Integrator/1
  Sum/1 -> Product/1
  Linv/1 -> Product1/1
  Vdq/1 -> Vector Concatenate/1
  Constant1/1 -> Vector Concatenate/2
  Vector Concatenate/1 -> Sum1/1

== system VIENA_part4/Subsystem/Induction Motor/Subsystem/Induction Machine Model/W Matrix Computation ==
  note: computes W(dPsi/dt)=[0                     -d(theta_s)/dt          0                       0;
      |                                     d(theta_s)/dt           0                      0                      0;
      |                                    0                              0                      0             -d(theta_r)/dt;
      |                                    0                              0             d(theta_r)/dt              0;]
  w_ref : Inport
  wm : Inport  Port=2
  Gain : Gain  Gain=Pp
  Gain1 : Gain  Gain=-1  SaturateOnIntegerOverflow=on  OutDataTypeStr=Inherit: Same as input  ParamDataTypeStr=Inherit: Same as input
  Product : Product
  Sum2 : Sum  Inputs=-+|  InputSameDT=on  SaturateOnIntegerOverflow=on  OutDataTypeStr=Inherit: Same as first input
  W(3,4)=wr-1 : Assignment  NumberOfDimensions=2  IndexOptions=Index vector (dialog),Index vector (dialog)  Indices=3,4  OutputSizes=1,1
  W(4,3)=1-wr1 : Assignment  NumberOfDimensions=2  IndexOptions=Index vector (dialog),Index vector (dialog)  Indices=4,3  OutputSizes=1,1
  u1 : Constant  Value="[ 0 -1  0  0; 1  0  0  0;  0  0  0  0;  0  0  0  0]"
  W : Outport  InitialOutput=0  VectorParamsAs1DForOutWhenUnconnected=off
  wires:
  Gain1/1 -> W(3,4)=wr-1/2
  W(3,4)=wr-1/1 -> W/1
  Sum2/1 -> W(4,3)=1-wr1/2, Gain1/1  "we-w"
  wm/1 -> Gain/1
  W(4,3)=1-wr1/1 -> W(3,4)=wr-1/1
  Gain/1 -> Sum2/1
  w_ref/1 -> Product/1, Sum2/2
  u1/1 -> Product/2
  Product/1 -> W(4,3)=1-wr1/1

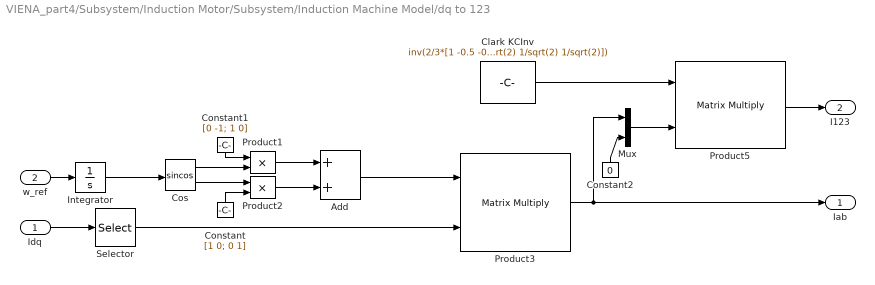
== system VIENA_part4/Subsystem/Induction Motor/Subsystem/Induction Machine Model/dq to 123 ==
  Idq : Inport
  w_ref : Inport  Port=2
  Add : Sum
  Clark KCInv : Constant  Value=inv(2/3*[1 -0.5 -0.5; 0 sqrt(3)/2 -sqrt(3)/2; 1/sqrt(2) 1/sqrt(2) 1/sqrt(2)])
  Constant : Constant  Value=[1 0; 0 1]
  Constant1 : Constant  Value=[0 -1; 1 0]
  Constant2 : Constant  Value=0
  Cos : Trigonometry  Operator=sincos
  Integrator : Integrator
  Mux : Mux  Inputs=2
  Product1 : Product
  Product2 : Product
  Product3 : Product  Multiplication=Matrix(*)
  Product5 : Product  Multiplication=Matrix(*)
  Selector : Selector  InputPortWidth=4  IndexOptions=Index vector (dialog)  Indices=[1 2]  OutputSizes=1
  Iab : Outport  VectorParamsAs1DForOutWhenUnconnected=off
  I123 : Outport  Port=2  VectorParamsAs1DForOutWhenUnconnected=off
  wires:
  Cos/1 -> Product1/2
  Constant1/1 -> Product1/1
  Product2/1 -> Add/2
  Cos/2 -> Product2/1
  Product1/1 -> Add/1
  Constant/1 -> Product2/2
  Add/1 -> Product3/1
  Idq/1 -> Selector/1
  Product3/1 -> Mux/1, Iab/1
  Clark KCInv/1 -> Product5/1
  Product5/1 -> I123/1
  Mux/1 -> Product5/2
  Constant2/1 -> Mux/2
  Selector/1 -> Product3/2
  Integrator/1 -> Cos/1
  w_ref/1 -> Integrator/1

== matlab function VIENA_part4/Subsystem/Car Dynamics/x-simplified model vehicle+wheel/MATLAB Troll ==
  data: u input; y output
function y = fTout(u)
y=0;
vx=u(1);
Troll=u(2);

if vx>0.01
   y=-Troll; % se o carro estiver a andar para a frente, este atrito trava o movimento
elseif vx<-0.01
    y=Troll; % se o carro estiver a andar para trás, este atrito trava o movimento
else
    y=0;
end

== matlab function VIENA_part4/Subsystem1/Control steering (with fixed frequency)/cria look_ahead ==
  data: map input; y1 output; y2 output; path_index input
function [y1,y2] = fcn(map,path_index)

coder.extrinsic('vecnorm')

y2=0;
path_look_ahead=3;
N=length(map);

window = zeros(path_look_ahead+1,2);

for i=1:path_look_ahead+1
    if path_index+i-1>N
        window(i,:)=map(min(path_index+i-1,N),:);
    else
        window(i,:)=map(path_index+i-1,:);
    end
    
end

y1=window;

if path_index==N
    y2=1;
end

== matlab function VIENA_part4/Subsystem1/Control steering (with fixed frequency)/compute diff angle ==
  data: zone input; y output; x input; y input; psi input
function y = fcn(zone,x,y,psi)

car_direction_vector=[-sin(psi) cos(psi)];
look_ahead_vector=[(zone(end,1)-x),zone(end,2)-y];
angle_car = atan2(car_direction_vector(2),car_direction_vector(1));
angle_look_ahead = atan2(look_ahead_vector(2),look_ahead_vector(1));



angle_diff = (angle_look_ahead-angle_car);
while angle_diff>pi
    angle_diff=angle_diff-2*pi;
end
while angle_diff<-pi
    angle_diff=angle_diff+2*pi;
end
y= angle_diff;

== matlab function VIENA_part4/Subsystem1/Control steering (with fixed frequency)/find index ==
  data: u input; y output; x input; y input
function y = fcn(u,x,y)

coder.extrinsic('vecnorm')
map=u;

[~, path_index]=min(vecnorm(map-repmat([x y],length(map),1),2,2));

y= path_index;
